simulink model "ref3ma_test"  (Simulink 4.00)
settings: Solver=FixedStepDiscrete  StartTime=0.0  StopTime=100.0  FixedStep=.001  RelTol=1e-3
settings Model: Creator=root  LastModifiedBy=root  SaveFormat=Structure  MaxDataPoints=10000  RTWSystemTargetFile=wintarget.tlc  RTWOptions="-aEnforceIntegerDowncast=1 -aExtMode=1 -aFoldNonRolledExpr=1 -aForceParamTrailComments=0 -aGenerateComments=1 -aIncHierarchyInIds=0 -aInlineInvariantSignals=0 -aInlineParameters=0 -aLocalBlockOutputs=1 -aLogVarNameModifier=\"rt_\" -aRTWVerbose=1 -aRollThreshold=5 -aShowEliminatedStatements=1"  RTWTemplateMakefile=wt_default_tmf  ExtModeAutoUpdateStatusClock=off

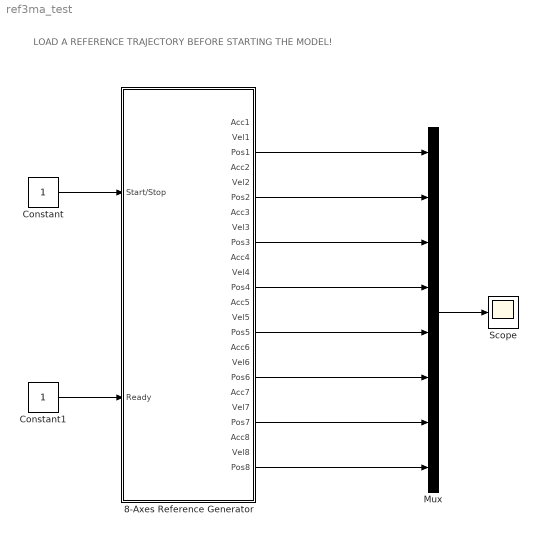
== system ref3ma_test ==
  note: LOAD A REFERENCE TRAJECTORY BEFORE STARTING THE MODEL!
  8-Axes Reference Generator : Subsystem
      settings: OpenFcn=global ref_part1 ref_part2 ref_part3 ref_part4 ref_part5 ref_part6 ref_part7 ref_part8; R12_r3g_axes  RTWFcnNameOpts=Auto  RTWFileNameOpts=Auto
  Constant : Constant  Value=1
  Constant1 : Constant  Value=1
  Mux : Mux  Inputs=8
  Scope : Scope
      settings: TimeRange=auto  YMin=-0.1  YMax=1.1  SaveToWorkspace=off  SaveName=ScopeData  LimitDataPoints=on  MaxDataPoints=5000
  wires:
  Constant1/1 -> 8-Axes Reference Generator/2(Ready)
  Constant/1 -> 8-Axes Reference Generator/1(Start/Stop)
  Mux/1 -> Scope/1
  8-Axes Reference Generator/3(Pos1) -> Mux/1
  8-Axes Reference Generator/6(Pos2) -> Mux/2
  8-Axes Reference Generator/9(Pos3) -> Mux/3
  8-Axes Reference Generator/12(Pos4) -> Mux/4
  8-Axes Reference Generator/15(Pos5) -> Mux/5
  8-Axes Reference Generator/18(Pos6) -> Mux/6
  8-Axes Reference Generator/21(Pos7) -> Mux/7
  8-Axes Reference Generator/24(Pos8) -> Mux/8

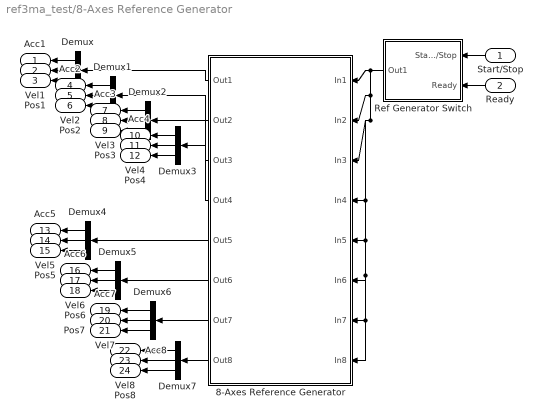
== system ref3ma_test/8-Axes Reference Generator ==
  Start/Stop : Inport  Orientation=left  Port=1  LatchInput=off
  Ready : Inport  Orientation=left  Port=2  LatchInput=off
  8-Axes Reference Generator : Subsystem  Orientation=left
      settings: OpenFcn=global ref_part1 ref_part2 ref_part3 ref_part4; r3g_axes  RTWFcnNameOpts=Auto  RTWFileNameOpts=Auto
      mask Type: 4-Axes Ref3 Block
  Demux{,1..7} (8 alike) : Demux  Orientation=left  Outputs=3  BusSelectionMode=off
  Ref Generator Switch : Subsystem  Orientation=left
      settings: RTWFcnNameOpts=Auto  RTWFileNameOpts=Auto
  Acc1 : Outport  Orientation=left  Port=1
  Vel1 : Outport  Orientation=left  Port=2
  Pos1 : Outport  Orientation=left  Port=3
  Acc2 : Outport  Orientation=left  Port=4
  Vel2 : Outport  Orientation=left  Port=5
  Pos2 : Outport  Orientation=left  Port=6
  Acc3 : Outport  Orientation=left  Port=7
  Vel3 : Outport  Orientation=left  Port=8
  Pos3 : Outport  Orientation=left  Port=9
  Acc4 : Outport  Orientation=left  Port=10
  Vel4 : Outport  Orientation=left  Port=11
  Pos4 : Outport  Orientation=left  Port=12
  Acc5 : Outport  Orientation=left  Port=13
  Vel5 : Outport  Orientation=left  Port=14
  Pos5 : Outport  Orientation=left  Port=15
  Acc6 : Outport  Orientation=left  Port=16
  Vel6 : Outport  Orientation=left  Port=17
  Pos6 : Outport  Orientation=left  Port=18
  Acc7 : Outport  Orientation=left  Port=19
  Vel7 : Outport  Orientation=left  Port=20
  Pos7 : Outport  Orientation=left  Port=21
  Acc8 : Outport  Orientation=left  Port=22
  Vel8 : Outport  Orientation=left  Port=23
  Pos8 : Outport  Orientation=left  Port=24
  wires:
  Demux3/3 -> Pos4/1
  Demux3/2 -> Vel4/1
  Demux3/1 -> Acc4/1
  Demux2/3 -> Pos3/1
  Demux2/2 -> Vel3/1
  Demux2/1 -> Acc3/1
  Demux1/3 -> Pos2/1
  Demux1/2 -> Vel2/1
  Demux1/1 -> Acc2/1
  Ready/1 -> Ref Generator Switch/2(Ready)
  Demux/3 -> Pos1/1
  Demux/2 -> Vel1/1
  Demux/1 -> Acc1/1
  Start/Stop/1 -> Ref Generator Switch/1(Start/Stop)
  8-Axes Reference Generator/1(Out1) -> Demux/1
  8-Axes Reference Generator/2(Out2) -> Demux1/1
  8-Axes Reference Generator/3(Out3) -> Demux2/1
  8-Axes Reference Generator/4(Out4) -> Demux3/1
  Ref Generator Switch/1(Out1) -> 8-Axes Reference Generator/3(In3), 8-Axes Reference Generator/4(In4), 8-Axes Reference Generator/5(In5), 8-Axes Reference Generator/6(In6), 8-Axes Reference Generator/7(In7), 8-Axes Reference Generator/8(In8), 8-Axes Reference Generator/2(In2), 8-Axes Reference Generator/1(In1)
  Demux4/1 -> Acc5/1
  Demux4/2 -> Vel5/1
  Demux4/3 -> Pos5/1
  Demux5/1 -> Acc6/1
  Demux5/2 -> Vel6/1
  Demux5/3 -> Pos6/1
  Demux6/1 -> Acc7/1
  Demux6/2 -> Vel7/1
  Demux6/3 -> Pos7/1
  Demux7/1 -> Acc8/1
  Demux7/2 -> Vel8/1
  Demux7/3 -> Pos8/1
  8-Axes Reference Generator/5(Out5) -> Demux4/1
  8-Axes Reference Generator/6(Out6) -> Demux5/1
  8-Axes Reference Generator/7(Out7) -> Demux6/1
  8-Axes Reference Generator/8(Out8) -> Demux7/1

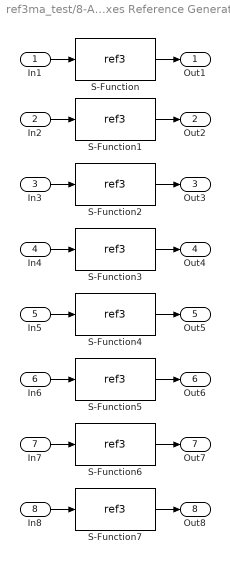
== system ref3ma_test/8-Axes Reference Generator/8-Axes Reference Generator ==
  In1 : Inport  Port=1  LatchInput=off
  In2 : Inport  Port=2  LatchInput=off
  In3 : Inport  Port=3  LatchInput=off
  In4 : Inport  Port=4  LatchInput=off
  In5 : Inport  Port=5  LatchInput=off
  In6 : Inport  Port=6  LatchInput=off
  In7 : Inport  Port=7  LatchInput=off
  In8 : Inport  Port=8  LatchInput=off
  S-Function : S-Function  FunctionName=ref3  Parameters=ref_part1  PortCounts=[]  SFunctionModules=''
  S-Function1 : S-Function  FunctionName=ref3  Parameters=ref_part2  PortCounts=[]  SFunctionModules=''
  S-Function2 : S-Function  FunctionName=ref3  Parameters=ref_part3  PortCounts=[]  SFunctionModules=''
  S-Function3 : S-Function  FunctionName=ref3  Parameters=ref_part4  PortCounts=[]  SFunctionModules=''
  S-Function4 : S-Function  FunctionName=ref3  Parameters=ref_part5  PortCounts=[]  SFunctionModules=''
  S-Function5 : S-Function  FunctionName=ref3  Parameters=ref_part6  PortCounts=[]  SFunctionModules=''
  S-Function6 : S-Function  FunctionName=ref3  Parameters=ref_part7  PortCounts=[]  SFunctionModules=''
  S-Function7 : S-Function  FunctionName=ref3  Parameters=ref_part8  PortCounts=[]  SFunctionModules=''
  Out1 : Outport  Port=1
  Out2 : Outport  Port=2
  Out3 : Outport  Port=3
  Out4 : Outport  Port=4
  Out5 : Outport  Port=5
  Out6 : Outport  Port=6
  Out7 : Outport  Port=7
  Out8 : Outport  Port=8
  wires:
  In4/1 -> S-Function3/1
  S-Function3/1 -> Out4/1
  In3/1 -> S-Function2/1
  S-Function2/1 -> Out3/1
  In2/1 -> S-Function1/1
  S-Function1/1 -> Out2/1
  In1/1 -> S-Function/1
  S-Function/1 -> Out1/1
  In5/1 -> S-Function4/1
  S-Function4/1 -> Out5/1
  In6/1 -> S-Function5/1
  S-Function5/1 -> Out6/1
  In7/1 -> S-Function6/1
  S-Function6/1 -> Out7/1
  In8/1 -> S-Function7/1
  S-Function7/1 -> Out8/1

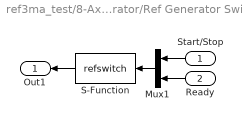
== system ref3ma_test/8-Axes Reference Generator/Ref Generator Switch ==
  Start/Stop : Inport  Orientation=left  Port=1  LatchInput=off
  Ready : Inport  Orientation=left  Port=2  LatchInput=off
  Mux1 : Mux  Orientation=left  Inputs=2
  S-Function : S-Function  Orientation=left  FunctionName=refswitch  PortCounts=[]  SFunctionModules=''
  Out1 : Outport  Orientation=left  Port=1
  wires:
  Ready/1 -> Mux1/2
  S-Function/1 -> Out1/1
  Start/Stop/1 -> Mux1/1
  Mux1/1 -> S-Function/1
